simulink model "Ass3_SISOclosed"  (Simulink 8.1)
settings: Solver=ode45  SolverMode=SingleTasking  StartTime=0.0  StopTime=T  RelTol=1e-3  AbsTol=1e-6
settings Model: Creator=schuurmans  LastModifiedBy=mpvlaar
settings DataIOCC: LimitDataPoints=off
settings OptimizationCC: BooleanDataType=off  InitFltsAndDblsToZero=on
settings DebuggingCC: SaveWithParameterizedLinksMsg=none  SignalResolutionControl=TryResolveAllWithWarning  SolverPrmCheckMsg=none  MultiTaskDSMMsg=warning  MultiTaskCondExecSysMsg=none  StrictBusMsg=None
settings HardwareCC: TargetUnknown=on
settings RTWCC: IncludeERTFirstTime=on
settings CodeAppCC: IgnoreCustomStorageClasses=off
settings GRTTargetCC: TargetFcnLib=ansi_tfl_tmw.mat  ModelReferenceCompliant=off  MatFileLogging=off

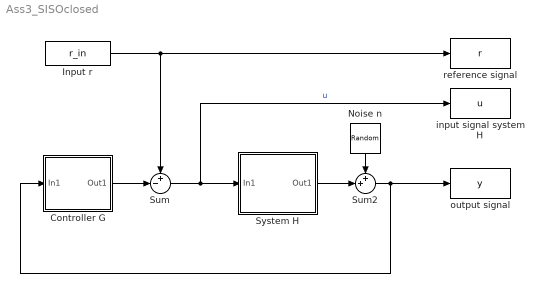
== system Ass3_SISOclosed ==
  Controller G : Subsystem
  Input r : FromWorkspace  VariableName=r_in  SampleTime=0
  Noise n : RandomNumber  Variance=.1  Seed=1465  SampleTime=0.01
  Sum : Sum  Inputs=+-|  SaturateOnIntegerOverflow=on  InputSameDT=on  OutDataTypeStr=Inherit: Same as first input
  Sum2 : Sum  Inputs=++|  SaturateOnIntegerOverflow=on  InputSameDT=on  OutDataTypeStr=Inherit: Same as first input
  System H : Subsystem
  input signal system H : ToWorkspace  VariableName=u  SampleTime=0.01
  output signal : ToWorkspace  VariableName=y  SampleTime=0.01
  reference signal : ToWorkspace  VariableName=r  SampleTime=0.01
  wires:
  Controller G/1(Out1) -> Sum/2
  Sum/1 -> System H/1(In1), input signal system H/1  "u"
  Noise n/1 -> Sum2/1
  System H/1(Out1) -> Sum2/2
  Sum2/1 -> output signal/1, Controller G/1(In1)
  Input r/1 -> reference signal/1, Sum/1

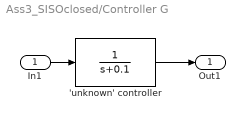
== system Ass3_SISOclosed/Controller G ==
  In1 : Inport
  'unknown' controller : TransferFcn  Denominator=[1 0.1]
  Out1 : Outport  InitialOutput=0
  wires:
  In1/1 -> 'unknown' controller/1
  'unknown' controller/1 -> Out1/1

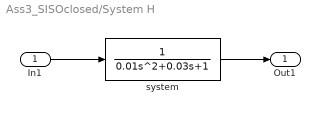
== system Ass3_SISOclosed/System H ==
  In1 : Inport
  system : TransferFcn  Numerator=1  Denominator=[0.01 0.03 1]
  Out1 : Outport  InitialOutput=0
  wires:
  In1/1 -> system/1
  system/1 -> Out1/1
